simulink model "Drone_simulation"  (R2024b)
settings: Solver=VariableStepAuto  StartTime=0.0  StopTime=t_stop  RelTol=1e-3
model workspace: external: MATLAB File Drone_parameters.m (data not in the file)
values from neighbouring files (symbols this model uses):
  d = 0.20    (= 0.2)    [Drone_parameters.m]
  disturbances_enabled = 0    [Drone_parameters.m]
  flight_mode = 3    [Drone_parameters.m]
  Fx_gust = 1.0    (= 1)    [Drone_parameters.m]
  Fy_gust = 1.0    (= 1)    [Drone_parameters.m]
  Fz_gust = 0.5    [Drone_parameters.m]
  inv_m = 0.3846    [Drone_parameters.m]
  Ixx = 0.05    [Drone_parameters.m]
  Iyy = 0.05    [Drone_parameters.m]
  Izz = 0.10    (= 0.1)    [Drone_parameters.m]
  Kd_phi = 0.5    [Drone_parameters.m]
  Kd_psi = 0.5    [Drone_parameters.m]
  Kd_theta = 0.28    [Drone_parameters.m]
  Kd_x = 0.16    [Drone_parameters.m]
  Kd_y = 0.16    [Drone_parameters.m]
  Kd_z = 4.5    [Drone_parameters.m]
  kf = 4.0e-5    (= 4e-05)    [Drone_parameters.m]
  Ki_phi = 0    [Drone_parameters.m]
  Ki_psi = 0    [Drone_parameters.m]
  Ki_theta = 0.28    [Drone_parameters.m]
  Ki_x = 0    [Drone_parameters.m]
  Ki_y = 0    [Drone_parameters.m]
  Ki_z = 0    [Drone_parameters.m]
  km = 1.0e-6    (= 1e-06)    [Drone_parameters.m]
  Kp_phi = 1.0    (= 1)    [Drone_parameters.m]
  Kp_psi = 1.0    (= 1)    [Drone_parameters.m]
  Kp_theta = 0.8    [Drone_parameters.m]
  Kp_x = 0.1    [Drone_parameters.m]
  Kp_y = 0.1    [Drone_parameters.m]
  Kp_z = 1.0    (= 1)    [Drone_parameters.m]
  mg = 25.5    [Drone_parameters.m]
  N_phi = 100    [Drone_parameters.m]
  N_psi = 100    [Drone_parameters.m]
  N_theta = 100    [Drone_parameters.m]
  N_x = 100    [Drone_parameters.m]
  N_y = 100    [Drone_parameters.m]
  N_z = 100    [Drone_parameters.m]
  omega_init = 399    [Drone_parameters.m]
  phi0 = 0    [Drone_parameters.m]
  phi_dot0 = 0    [Drone_parameters.m]
  phi_manual = 0    [Drone_parameters.m]
  pitch_pair_allocation = 1/(2*d)    (= 2.5)    [Drone_parameters.m]
  psi0 = 0    [Drone_parameters.m]
  psi_des = deg2rad(0)    [Drone_parameters.m]
  psi_dot0 = 0    [Drone_parameters.m]
  psi_hold = 0    [Drone_parameters.m]
  psi_manual = 0    [Drone_parameters.m]
  rad_to_deg = 180/pi    (= 57.2957795131)    [Drone_parameters.m]
  replay_collective_to_pair_thrust_N = 51.0    (= 51)    [Drone_parameters.m]
  replay_enabled = 0    [Drone_parameters.m]
  roll_motor_allocation = 1/(4*d)    (= 1.25)    [Drone_parameters.m]
  seed_phi = 104    [Drone_parameters.m]
  seed_psi = 106    [Drone_parameters.m]
  seed_theta = 105    [Drone_parameters.m]
  seed_x = 101    [Drone_parameters.m]
  seed_y = 102    [Drone_parameters.m]
  seed_z = 103    [Drone_parameters.m]
  sensor_noise_enabled = 0    [Drone_parameters.m]
  sensor_noise_tau_attitude = 0.10    (= 0.1)    [Drone_parameters.m]
  sensor_noise_tau_position = 0.20    (= 0.2)    [Drone_parameters.m]
  sensor_sample_time = 0.02    [Drone_parameters.m]
  sigma_phi = deg2rad(0.02)    [Drone_parameters.m]
  sigma_psi = deg2rad(0.05)    [Drone_parameters.m]
  sigma_theta = deg2rad(0.02)    [Drone_parameters.m]
  sigma_x = 0.002    [Drone_parameters.m]
  sigma_y = 0.002    [Drone_parameters.m]
  sigma_z = 0.001    [Drone_parameters.m]
  t_Fx_end = 11    [Drone_parameters.m]
  t_Fx_start = 10    [Drone_parameters.m]
  t_Fy_end = 16    [Drone_parameters.m]
  t_Fy_start = 15    [Drone_parameters.m]
  t_Fz_end = 21    [Drone_parameters.m]
  t_Fz_start = 20    [Drone_parameters.m]
  t_pitch_end = 30.5    [Drone_parameters.m]
  t_pitch_start = 30    [Drone_parameters.m]
  t_roll_end = 25.5    [Drone_parameters.m]
  t_roll_start = 25    [Drone_parameters.m]
  t_step_xy = 1    [Drone_parameters.m]
  t_step_yaw = 1    [Drone_parameters.m]
  t_step_z = 0    [Drone_parameters.m]
  t_yaw_end = 35.5    [Drone_parameters.m]
  t_yaw_start = 35    [Drone_parameters.m]
  tau_m = 0.05    [Drone_parameters.m]
  tau_pitch_gust = 0.01    [Drone_parameters.m]
  tau_roll_gust = 0.01    [Drone_parameters.m]
  tau_yaw_gust = 0.002    [Drone_parameters.m]
  theta0 = 0    [Drone_parameters.m]
  theta_dot0 = 0    [Drone_parameters.m]
  theta_manual = 0    [Drone_parameters.m]
  tilt_max = 0.1745    [Drone_parameters.m]
  Tmax = 12.5    [Drone_parameters.m]
  Tmin = 0    [Drone_parameters.m]
  vx0 = 0    [Drone_parameters.m]
  vy0 = 0    [Drone_parameters.m]
  vz0 = 0    [Drone_parameters.m]
  x0 = 0    [Drone_parameters.m]
  x_des = 4    [Drone_parameters.m]
  x_hold = 0    [Drone_parameters.m]
  x_manual = 0    [Drone_parameters.m]
  y0 = 0    [Drone_parameters.m]
  y_des = 2    [Drone_parameters.m]
  y_hold = 0    [Drone_parameters.m]
  y_manual = 0    [Drone_parameters.m]
  yaw_motor_allocation = kf/(4*km)    (= 10)    [Drone_parameters.m]
  z0 = 0    [Drone_parameters.m]
  z_des = 1    [Drone_parameters.m]
  z_hold = 1    [Drone_parameters.m]
  z_manual = 1    [Drone_parameters.m]
libraries: slpidlib x6
(part 1 of 2)
settings Model: Creator=shiyu  LastModifiedBy=shiyu

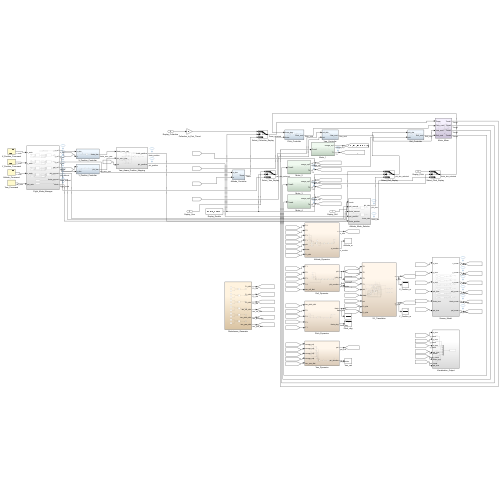
[thumbnail: Simulink's stored preview of the top-level diagram]
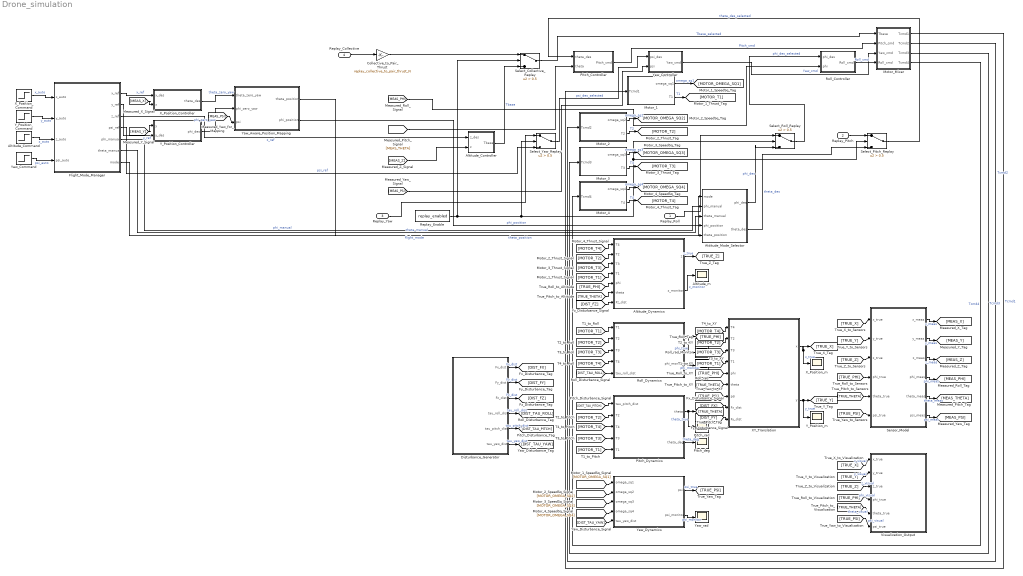
== system Drone_simulation ==
  Replay_Roll : Inport
  Replay_Pitch : Inport  Port=2
  Replay_Yaw : Inport  Port=3
  Replay_Collective : Inport  Port=4
  Altitude_Command : Step  Time=t_step_z  After=z_des  SampleTime=0
  Altitude_Controller : Subsystem  Description=Altitude error -> PID -> pair thrust correction + pair hover feed-forward. Tbase is thrust per motor pair (N).
  Altitude_Dynamics : Subsystem  Description=Inputs in unchanged port order: T4,T2,T3,T1 (N), phi,theta (rad). Both outputs are altitude (m); z_monitor duplicates z.
  Altitude_m : Scope
  Attitude_Mode_Selector : Subsystem
  Collective_to_Pair_Thrust : Gain  Gain=replay_collective_to_pair_thrust_N
  Disturbance_Generator : Subsystem  Description=Six switchable finite pulses. Outputs are world-frame forces Fx/Fy/Fz (N) and roll/pitch/yaw disturbance torques (N*m). Set disturbances_enabled=0 or 1 in Drone_parameters.m.
  Flight_Mode_Manager : Subsystem
  Motor_1 : Subsystem  Description=Motor 1: command Tcmd1 (N); output 1 omega_sq1 ((rad/s)^2), output 2 T1 (N). Rotor-speed lag and initialization preserved.
  Motor_2 : Subsystem  Description=Motor 2: command Tcmd2 (N); output 1 omega_sq2 ((rad/s)^2), output 2 T2 (N).
  Motor_3 : Subsystem  Description=Motor 3: command Tcmd3 (N); output 1 omega_sq3 ((rad/s)^2), output 2 T3 (N).
  Motor_4 : Subsystem  Description=Motor 4: command Tcmd4 (N); output 1 omega_sq4 ((rad/s)^2), output 2 T4 (N). Former Psi output was speed squared, not yaw.
  Motor_Mixer : Subsystem  Description=Input order: Tbase, Pitch_cmd, Yaw_cmd, Roll_cmd. Outputs Tcmd1..4 (N). Existing M1/M2 pair uses Tbase + Pitch_cmd; M3/M4 uses Tbase - Pitch_cmd. Do not change signs during cosmetic cleanup.
  Pitch_Controller : Subsystem  Description=Pitch angle error (rad) -> PID -> pitch pair thrust correction (N). Existing mixer sign and scaling preserved.
  Pitch_Dynamics : Subsystem  Description=Inputs: disturbance torque (N m), T2,T4,T3,T1 (N). Outputs: theta (rad), theta_deg (deg). Independent Euler-angle double integrator.
  Pitch_deg : Scope
  Pitch_rad : Scope
  Replay_Enable : Constant  Value=replay_enabled
  Roll_Controller : Subsystem  Description=Roll angle error (rad) -> PID -> per-motor differential thrust correction (N).
  Roll_Dynamics : Subsystem  Description=Inputs T1,T2,T3,T4 (N). Both outputs are roll angle (rad); phi_monitor duplicates phi. Independent Euler-angle double integrator.
  Roll_rad : Scope
  Roll_rad_Monitor : Scope
  Select_Collective_Replay : Switch  Criteria=u2 > Threshold  Threshold=0.5  SaturateOnIntegerOverflow=off  InputSameDT=off
  Select_Pitch_Replay : Switch  Criteria=u2 > Threshold  Threshold=0.5  SaturateOnIntegerOverflow=off  InputSameDT=off
  Select_Roll_Replay : Switch  Criteria=u2 > Threshold  Threshold=0.5  SaturateOnIntegerOverflow=off  InputSameDT=off
  Select_Yaw_Replay : Switch  Criteria=u2 > Threshold  Threshold=0.5  SaturateOnIntegerOverflow=off  InputSameDT=off
  Sensor_Model : Subsystem
  Visualization_Output : Subsystem
  XY_Translation : Subsystem  Description=Inputs: T4,T2,T3,T1 (N), phi,theta,psi (rad). Outputs x,y (m). Implements the ZYX body-z thrust direction: Fx/T = cos(psi)*sin(theta)*cos(phi) + sin(psi)*sin(phi); Fy/T = sin(psi)*sin(theta)*cos(phi) - cos(psi)*sin(phi). Corrected and validated 2026-09-03.
  X_Position_Command : Step  Time=t_step_xy  After=x_des  SampleTime=0
  X_Position_Controller : Subsystem  Description=x_des - x (m) -> existing PD -> pitch command limit (rad).
  X_Position_m : Scope
  Y_Position_Command : Step  Time=t_step_xy  After=y_des  SampleTime=0
  Y_Position_Controller : Subsystem  Description=Input order preserved: port 1 is actual y; port 2 is y_des. Error y_des - y, followed by existing negative roll-command sign.
  Y_Position_m : Scope
  Yaw_Aware_Position_Mapping : Subsystem
  Yaw_Command : Step  Time=t_step_yaw  After=psi_des  SampleTime=0
  Yaw_Controller : Subsystem  Description=Yaw angle error (rad) -> PID -> per-motor differential thrust correction (N).
  Yaw_Dynamics : Subsystem  Description=Inputs omega_sq1..4 ((rad/s)^2); reaction-torque coefficients are applied inside. Both outputs are yaw angle (rad); psi_monitor duplicates psi.
  Yaw_rad : Scope
  wires:
  Motor_2/1(omega_sq2) -> [MOTOR_OMEGA_SQ2]  "omega_sq2"
  Altitude_Dynamics/2(z_monitor) -> Altitude_m/1  "z_monitor"
  Roll_Dynamics/2(phi_monitor) -> Roll_rad/1  "phi_monitor"
  Yaw_Dynamics/2(psi_monitor) -> Yaw_rad/1  "psi_monitor"
  Motor_3/2(T3) -> [MOTOR_T3]  "T3"
  Pitch_Dynamics/2(theta_deg) -> Pitch_deg/1  "theta_deg"
  Motor_3/1(omega_sq3) -> [MOTOR_OMEGA_SQ3]  "omega_sq3"
  Motor_2/2(T2) -> [MOTOR_T2]  "T2"
  Flight_Mode_Manager/2(y_ref) -> Y_Position_Controller/2(y_des)  "y_ref"
  Flight_Mode_Manager/1(x_ref) -> X_Position_Controller/1(x_des)  "x_ref"
  Sensor_Model/6(psi_meas) -> [MEAS_PSI]  "psi_meas"
  Sensor_Model/5(theta_meas) -> [MEAS_THETA]  "theta_meas"
  Sensor_Model/4(phi_meas) -> [MEAS_PHI]  "phi_meas"
  Sensor_Model/3(z_meas) -> [MEAS_Z]  "z_meas"
  Sensor_Model/2(y_meas) -> [MEAS_Y]  "y_meas"
  Sensor_Model/1(x_meas) -> [MEAS_X]  "x_meas"
  Motor_4/2(T4) -> [MOTOR_T4]  "T4"
  Roll_Dynamics/1(phi) -> [TRUE_PHI], Roll_rad_Monitor/1  "phi_true"
  Pitch_Dynamics/1(theta) -> [TRUE_THETA], Pitch_rad/1  "theta_true"
  XY_Translation/1(x) -> [TRUE_X], X_Position_m/1  "x_true"
  XY_Translation/2(y) -> [TRUE_Y], Y_Position_m/1  "y_true"
  Yaw_Dynamics/1(psi) -> [TRUE_PSI]  "psi_true"
  Disturbance_Generator/1(Fx_dist) -> [DIST_FX]  "Fx_dist"
  Disturbance_Generator/2(Fy_dist) -> [DIST_FY]  "Fy_dist"
  Disturbance_Generator/3(Fz_dist) -> [DIST_FZ]  "Fz_dist"
  Disturbance_Generator/4(tau_roll_dist) -> [DIST_TAU_ROLL]  "tau_roll_dist"
  Disturbance_Generator/5(tau_pitch_dist) -> [DIST_TAU_PITCH]  "tau_pitch_dist"
  Disturbance_Generator/6(tau_yaw_dist) -> [DIST_TAU_YAW]  "tau_yaw_dist"
  X_Position_Controller/1(theta_des) -> Yaw_Aware_Position_Mapping/1(theta_zero_yaw)  "theta_zero_yaw"
  X_Position_Command/1 -> Flight_Mode_Manager/1(x_auto)  "x_auto"
  Y_Position_Controller/1(phi_des) -> Yaw_Aware_Position_Mapping/2(phi_zero_yaw)  "phi_zero_yaw"
  Y_Position_Command/1 -> Flight_Mode_Manager/2(y_auto)  "y_auto"
  Motor_4/1(omega_sq4) -> [MOTOR_OMEGA_SQ4]  "omega_sq4"
  Altitude_Dynamics/1(z) -> [TRUE_Z]  "z_true"
  Yaw_Command/1 -> Flight_Mode_Manager/4(psi_auto)  "psi_auto"
  Altitude_Command/1 -> Flight_Mode_Manager/3(z_auto)  "z_auto"
  [MEAS_X] -> X_Position_Controller/2(x)
  [MEAS_Y] -> Y_Position_Controller/1(y)
  [MOTOR_T1] -> Altitude_Dynamics/4(T1)
  [MOTOR_T2] -> Altitude_Dynamics/2(T2)
  [MOTOR_T3] -> Altitude_Dynamics/3(T3)
  [MOTOR_T4] -> Altitude_Dynamics/1(T4)
  [MOTOR_OMEGA_SQ1] -> Yaw_Dynamics/1(omega_sq1)
  [MOTOR_OMEGA_SQ2] -> Yaw_Dynamics/2(omega_sq2)
  [MOTOR_OMEGA_SQ3] -> Yaw_Dynamics/3(omega_sq3)
  [MOTOR_OMEGA_SQ4] -> Yaw_Dynamics/4(omega_sq4)
  [MEAS_PSI] -> Yaw_Aware_Position_Mapping/3(psi)
  [MOTOR_T4] -> XY_Translation/1(T4)
  [MOTOR_T4] -> Pitch_Dynamics/3(T4)
  [MOTOR_T4] -> Roll_Dynamics/4(T4)
  [MOTOR_T3] -> XY_Translation/3(T3)
  [MOTOR_T3] -> Pitch_Dynamics/4(T3)
  [MOTOR_T3] -> Roll_Dynamics/3(T3)
  [MOTOR_T2] -> XY_Translation/2(T2)
  [MOTOR_T2] -> Pitch_Dynamics/2(T2)
  [MOTOR_T2] -> Roll_Dynamics/2(T2)
  [MOTOR_T1] -> XY_Translation/4(T1)
  [MOTOR_T1] -> Pitch_Dynamics/5(T1)
  [MOTOR_T1] -> Roll_Dynamics/1(T1)
  [TRUE_X] -> Sensor_Model/1(x_true)
  [TRUE_Y] -> Sensor_Model/2(y_true)
  [TRUE_Z] -> Sensor_Model/3(z_true)
  [TRUE_PHI] -> Sensor_Model/4(phi_true)
  [TRUE_THETA] -> Sensor_Model/5(theta_true)
  [TRUE_PSI] -> Sensor_Model/6(psi_true)
  [TRUE_PHI] -> Altitude_Dynamics/5(phi)
  [TRUE_PHI] -> XY_Translation/5(phi)
  [TRUE_THETA] -> Altitude_Dynamics/6(theta)
  [TRUE_THETA] -> XY_Translation/6(theta)
  [TRUE_PSI] -> XY_Translation/7(psi)
  [DIST_FX] -> XY_Translation/8(Fx_dist)
  [DIST_FY] -> XY_Translation/9(Fy_dist)
  [DIST_FZ] -> Altitude_Dynamics/7(Fz_dist)
  [DIST_TAU_ROLL] -> Roll_Dynamics/5(tau_roll_dist)
  [DIST_TAU_PITCH] -> Pitch_Dynamics/1(tau_pitch_dist)
  [DIST_TAU_YAW] -> Yaw_Dynamics/5(tau_yaw_dist)
  [TRUE_PSI] -> Visualization_Output/6(psi_true)  "psi_visual"
  [TRUE_THETA] -> Visualization_Output/5(theta_true)  "theta_visual"
  [TRUE_PHI] -> Visualization_Output/4(phi_true)  "phi_visual"
  [TRUE_Z] -> Visualization_Output/3(z_true)  "z_visual"
  [TRUE_Y] -> Visualization_Output/2(y_true)  "y_visual"
  [TRUE_X] -> Visualization_Output/1(x_true)  "x_visual"
  Select_Collective_Replay/1 -> Motor_Mixer/1(Tbase)  "Tbase_selected"
  Altitude_Controller/1(Tbase) -> Select_Collective_Replay/3  "Tbase"
  Collective_to_Pair_Thrust/1 -> Select_Collective_Replay/1
  Replay_Collective/1 -> Collective_to_Pair_Thrust/1
  Select_Yaw_Replay/1 -> Yaw_Controller/1(psi_des)  "psi_des_selected"
  Replay_Yaw/1 -> Select_Yaw_Replay/1
  Flight_Mode_Manager/4(psi_ref) -> Select_Yaw_Replay/3  "psi_ref"
  Select_Pitch_Replay/1 -> Pitch_Controller/1(theta_des)  "theta_des_selected"
  Replay_Pitch/1 -> Select_Pitch_Replay/1
  Attitude_Mode_Selector/2(theta_des) -> Select_Pitch_Replay/3  "theta_des"
  Select_Roll_Replay/1 -> Roll_Controller/1(phi_des)  "phi_des_selected"
  Replay_Enable/1 -> Select_Pitch_Replay/2, Select_Roll_Replay/2, Select_Yaw_Replay/2, Select_Collective_Replay/2
  Replay_Roll/1 -> Select_Roll_Replay/1
  Attitude_Mode_Selector/1(phi_des) -> Select_Roll_Replay/3  "phi_des"
  [MEAS_PSI] -> Yaw_Controller/2(psi)
  [MEAS_THETA] -> Pitch_Controller/2(theta)
  [MEAS_PHI] -> Roll_Controller/2(phi)
  [MEAS_Z] -> Altitude_Controller/2(z)
  Pitch_Controller/1(Pitch_cmd) -> Motor_Mixer/2(Pitch_cmd)  "Pitch_cmd"
  Yaw_Controller/1(Yaw_cmd) -> Motor_Mixer/3(Yaw_cmd)  "Yaw_cmd"
  Motor_Mixer/4(Tcmd4) -> Motor_4/1(Tcmd4)  "Tcmd4"
  Roll_Controller/1(Roll_cmd) -> Motor_Mixer/4(Roll_cmd)  "Roll_cmd"
  Flight_Mode_Manager/3(z_ref) -> Altitude_Controller/1(z_des)  "z_ref"
  Flight_Mode_Manager/7(mode) -> Attitude_Mode_Selector/1(mode)  "flight_mode"
  Flight_Mode_Manager/5(phi_manual) -> Attitude_Mode_Selector/2(phi_manual)  "phi_manual"
  Flight_Mode_Manager/6(theta_manual) -> Attitude_Mode_Selector/3(theta_manual)  "theta_manual"
  Yaw_Aware_Position_Mapping/2(phi_position) -> Attitude_Mode_Selector/4(phi_position)  "phi_position"
  Yaw_Aware_Position_Mapping/1(theta_position) -> Attitude_Mode_Selector/5(theta_position)  "theta_position"
  Motor_Mixer/3(Tcmd3) -> Motor_3/1(Tcmd3)  "Tcmd3"
  Motor_1/2(T1) -> [MOTOR_T1]  "T1"
  Motor_Mixer/2(Tcmd2) -> Motor_2/1(Tcmd2)  "Tcmd2"
  Motor_Mixer/1(Tcmd1) -> Motor_1/1(Tcmd1)  "Tcmd1"
  Motor_1/1(omega_sq1) -> [MOTOR_OMEGA_SQ1]  "omega_sq1"

== system Drone_simulation/Altitude_Controller ==
  z_des : Inport
  z : Inport  Port=2
  Altitude_Error : Sum  Inputs=-+|
  Altitude_PID : slpidlib/PID Controller  Controller=PID  Form=Parallel  TimeDomain=Continuous-time  UseExternalTs=off  SampleTime=-1  IntegratorMethod=Forward Euler  FilterMethod=Forward Euler  ControllerParametersSource=internal  P=Kp_z  I=Ki_z  UseKiTs=off  D=Kd_z  UseExternalDerivativeSource=off  N=N_z  UseFilter=on  TunerSelectOption=Transfer Function Based (PID Tuner App)  InitialConditionSource=internal  InitialConditionForIntegrator=0  InitialConditionForFilter=0  DifferentiatorICPrevScaledInput=0  ExternalReset=none  TrackingMode=off  Kt=1  LimitOutput=off  SatLimitsSource=internal  UpperSaturationLimit=inf  LowerSaturationLimit=-inf  LinearizeAsGain=on  AntiWindupMode=none  Kb=1  LimitIntegrator=off  UpperIntegratorSaturationLimit=inf  LowerIntegratorSaturationLimit=-inf  POutMin=[]  POutMax=[]  IOutMin=[]  IOutMax=[]  DOutMin=[]  DOutMax=[]  NOutMin=[]  NOutMax=[]  SumOutMin=[]  SumOutMax=[]  SaturationOutMin=[]  SaturationOutMax=[]  PParamMin=[]  PParamMax=[]  IParamMin=[]  IParamMax=[]  DParamMin=[]  DParamMax=[]  NParamMin=[]  NParamMax=[]  KbParamMin=[]  KbParamMax=[]  KtParamMin=[]  KtParamMax=[]  KbOutMin=[]  KbOutMax=[]  KtOutMin=[]  KtOutMax=[]  IntegratorOutMin=[]  IntegratorOutMax=[]  FilterOutMin=[]  FilterOutMax=[]  SumI1OutMin=[]  SumI1OutMax=[]  SumI2OutMin=[]  SumI2OutMax=[]  SumI3OutMin=[]  SumI3OutMax=[]  SumI4OutMin=[]  SumI4OutMax=[]  SumDOutMin=[]  SumDOutMax=[]  DifferentiatorOutMin=[]  DifferentiatorOutMax=[]  FilterDiffOutCoefMin=[]  FilterDiffOutCoefMax=[]  ReciprocalOutMin=[]  ReciprocalOutMax=[]  SumDenOutMin=[]  SumDenOutMax=[]  SumNumOutMin=[]  SumNumOutMax=[]  DivideOutMin=[]  DivideOutMax=[]  UdiffTsProdOutMin=[]  UdiffTsProdOutMax=[]  NTsProdOutMin=[]  NTsProdOutMax=[]  UintegralTsProdOutMin=[]  UintegralTsProdOutMax=[]  UngainTsProdOutMin=[]  UngainTsProdOutMax=[]  ClampingZeroOutDataTypeStr=Inherit: Inherit via back propagation  ClampingZeroOutMin=[]  ClampingZeroOutMax=[]  FilterDenConstantOutDataTypeStr=Inherit: Inherit via back propagation  FilterDenConstantOutMin=[]  FilterDenConstantOutMax=[]  PCopyOutDataTypeStr=Inherit: Inherit via back propagation  PCopyOutMin=[]  PCopyOutMax=[]  NCopyOutDataTypeStr=Inherit: Inherit via back propagation  NCopyOutMin=[]  NCopyOutMax=[]  IntegratorContinuousStateAttributes=''  IntegratorStateMustResolveToSignalObject=off  IntegratorRTWStateStorageClass=Auto  FilterContinuousStateAttributes=''  FilterStateMustResolveToSignalObject=off  FilterRTWStateStorageClass=Auto  ParallelPVariant=InternalParameters  IdealPVariant=Disabled  IVariant=InternalParameters  DVariant=InternalParameters  IntegratorVariant=Continuous  SatVariant=Disabled  AWVariant=Passthrough  PCopyVariant=Disabled  TRVariant=Disabled  FdbkBlocksVariant=Forward  IdealPFdbkVariant=Disabled  SatFdbkVariant=Disabled  DerivativeFilterVariant=ContFilter  NVariant=InternalParameters  NCopyVariant=Disabled  FilterICVariant=InternalICsFilter  IntegratorICVariant=InternalICs  ExternalResetVariant=Disabled  TRSumVariant=Passthrough  SumFdbkVariant=Disabled  SumVariant=Sum_PID  TsampFilterVariant=InternalTs  TsampNgainVariant=Passthrough  TsampIntegralVariant=Disabled_SignalSpec  ExternalSaturationOutDataTypeStr=Inherit: Same as second input  DerivativeSourceVariant=ErrorSignal  PreIntVariant=InternalPreInt
  Pair_Collective_Command : Sum  Inputs=|++
  Pair_Hover_Thrust : Constant  Value=mg/2
  Total_To_Pair_Correction : Gain  Gain=0.5
  Tbase : Outport
  wires:
  z/1 -> Altitude_Error/1
  z_des/1 -> Altitude_Error/2
  Pair_Hover_Thrust/1 -> Pair_Collective_Command/2
  Pair_Collective_Command/1 -> Tbase/1
  Total_To_Pair_Correction/1 -> Pair_Collective_Command/1
  Altitude_PID/1 -> Total_To_Pair_Correction/1
  Altitude_Error/1 -> Altitude_PID/1

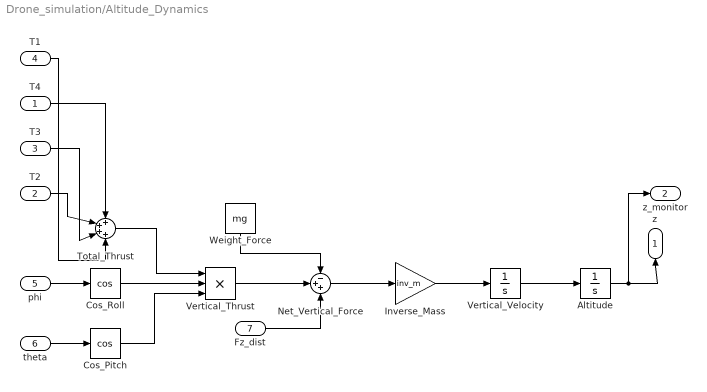
== system Drone_simulation/Altitude_Dynamics ==
  T4 : Inport
  T2 : Inport  Port=2
  T3 : Inport  Port=3
  T1 : Inport  Port=4
  phi : Inport  Port=5
  theta : Inport  Port=6
  Fz_dist : Inport  Port=7
  Altitude : Integrator  InitialCondition=z0
  Cos_Pitch : Trigonometry  Operator=cos
  Cos_Roll : Trigonometry  Operator=cos
  Inverse_Mass : Gain  Gain=inv_m
  Net_Vertical_Force : Sum  Inputs=-++
  Total_Thrust : Sum  Inputs=++++
  Vertical_Thrust : Product  Inputs=3
  Vertical_Velocity : Integrator  InitialCondition=vz0
  Weight_Force : Constant  Value=mg
  z : Outport
  z_monitor : Outport  Port=2
  wires:
  T1/1 -> Total_Thrust/4
  T2/1 -> Total_Thrust/2
  theta/1 -> Cos_Pitch/1
  Weight_Force/1 -> Net_Vertical_Force/1
  T4/1 -> Total_Thrust/1
  T3/1 -> Total_Thrust/3
  phi/1 -> Cos_Roll/1
  Total_Thrust/1 -> Vertical_Thrust/1
  Cos_Roll/1 -> Vertical_Thrust/2
  Cos_Pitch/1 -> Vertical_Thrust/3
  Altitude/1 -> z_monitor/1, z/1
  Vertical_Thrust/1 -> Net_Vertical_Force/2
  Net_Vertical_Force/1 -> Inverse_Mass/1
  Inverse_Mass/1 -> Vertical_Velocity/1
  Vertical_Velocity/1 -> Altitude/1
  Fz_dist/1 -> Net_Vertical_Force/3

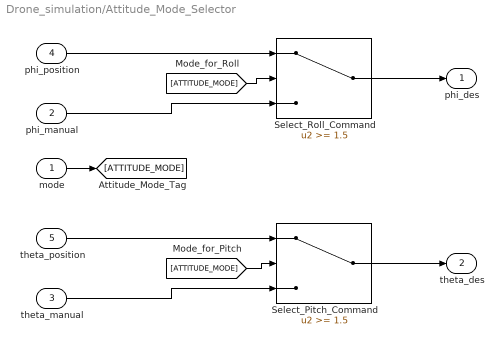
== system Drone_simulation/Attitude_Mode_Selector ==
  mode : Inport
  phi_manual : Inport  Port=2
  theta_manual : Inport  Port=3
  phi_position : Inport  Port=4
  theta_position : Inport  Port=5
  Select_Pitch_Command : Switch  Threshold=1.5  SaturateOnIntegerOverflow=off  InputSameDT=off
  Select_Roll_Command : Switch  Threshold=1.5  SaturateOnIntegerOverflow=off  InputSameDT=off
  phi_des : Outport
  theta_des : Outport  Port=2
  wires:
  [ATTITUDE_MODE] -> Select_Pitch_Command/2
  [ATTITUDE_MODE] -> Select_Roll_Command/2
  phi_position/1 -> Select_Roll_Command/1
  mode/1 -> [ATTITUDE_MODE]
  phi_manual/1 -> Select_Roll_Command/3
  Select_Roll_Command/1 -> phi_des/1
  theta_position/1 -> Select_Pitch_Command/1
  theta_manual/1 -> Select_Pitch_Command/3
  Select_Pitch_Command/1 -> theta_des/1

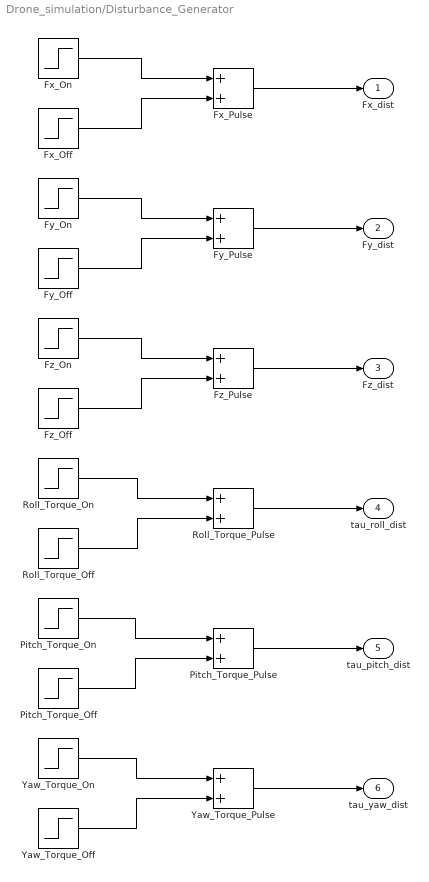
== system Drone_simulation/Disturbance_Generator ==
  Fx_Off : Step  Time=t_Fx_end  After=-disturbances_enabled*Fx_gust  SampleTime=0
  Fx_On : Step  Time=t_Fx_start  After=disturbances_enabled*Fx_gust  SampleTime=0
  Fx_Pulse : Sum
  Fy_Off : Step  Time=t_Fy_end  After=-disturbances_enabled*Fy_gust  SampleTime=0
  Fy_On : Step  Time=t_Fy_start  After=disturbances_enabled*Fy_gust  SampleTime=0
  Fy_Pulse : Sum
  Fz_Off : Step  Time=t_Fz_end  After=-disturbances_enabled*Fz_gust  SampleTime=0
  Fz_On : Step  Time=t_Fz_start  After=disturbances_enabled*Fz_gust  SampleTime=0
  Fz_Pulse : Sum
  Pitch_Torque_Off : Step  Time=t_pitch_end  After=-disturbances_enabled*tau_pitch_gust  SampleTime=0
  Pitch_Torque_On : Step  Time=t_pitch_start  After=disturbances_enabled*tau_pitch_gust  SampleTime=0
  Pitch_Torque_Pulse : Sum
  Roll_Torque_Off : Step  Time=t_roll_end  After=-disturbances_enabled*tau_roll_gust  SampleTime=0
  Roll_Torque_On : Step  Time=t_roll_start  After=disturbances_enabled*tau_roll_gust  SampleTime=0
  Roll_Torque_Pulse : Sum
  Yaw_Torque_Off : Step  Time=t_yaw_end  After=-disturbances_enabled*tau_yaw_gust  SampleTime=0
  Yaw_Torque_On : Step  Time=t_yaw_start  After=disturbances_enabled*tau_yaw_gust  SampleTime=0
  Yaw_Torque_Pulse : Sum
  Fx_dist : Outport
  Fy_dist : Outport  Port=2
  Fz_dist : Outport  Port=3
  tau_roll_dist : Outport  Port=4
  tau_pitch_dist : Outport  Port=5
  tau_yaw_dist : Outport  Port=6
  wires:
  Yaw_Torque_Pulse/1 -> tau_yaw_dist/1
  Yaw_Torque_Off/1 -> Yaw_Torque_Pulse/2
  Yaw_Torque_On/1 -> Yaw_Torque_Pulse/1
  Pitch_Torque_Pulse/1 -> tau_pitch_dist/1
  Pitch_Torque_Off/1 -> Pitch_Torque_Pulse/2
  Pitch_Torque_On/1 -> Pitch_Torque_Pulse/1
  Roll_Torque_Pulse/1 -> tau_roll_dist/1
  Roll_Torque_Off/1 -> Roll_Torque_Pulse/2
  Roll_Torque_On/1 -> Roll_Torque_Pulse/1
  Fz_Pulse/1 -> Fz_dist/1
  Fz_Off/1 -> Fz_Pulse/2
  Fz_On/1 -> Fz_Pulse/1
  Fy_Pulse/1 -> Fy_dist/1
  Fy_Off/1 -> Fy_Pulse/2
  Fy_On/1 -> Fy_Pulse/1
  Fx_Pulse/1 -> Fx_dist/1
  Fx_Off/1 -> Fx_Pulse/2
  Fx_On/1 -> Fx_Pulse/1

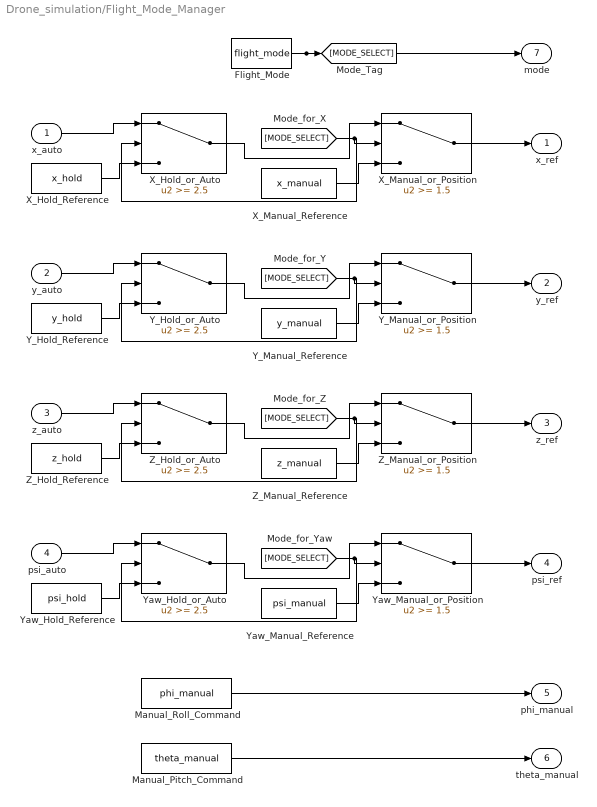
== system Drone_simulation/Flight_Mode_Manager ==
  x_auto : Inport
  y_auto : Inport  Port=2
  z_auto : Inport  Port=3
  psi_auto : Inport  Port=4
  Flight_Mode : Constant  Value=flight_mode
  Manual_Pitch_Command : Constant  Value=theta_manual
  Manual_Roll_Command : Constant  Value=phi_manual
  X_Hold_Reference : Constant  Value=x_hold
  X_Hold_or_Auto : Switch  Threshold=2.5  SaturateOnIntegerOverflow=off  InputSameDT=off
  X_Manual_Reference : Constant  Value=x_manual
  X_Manual_or_Position : Switch  Threshold=1.5  SaturateOnIntegerOverflow=off  InputSameDT=off
  Y_Hold_Reference : Constant  Value=y_hold
  Y_Hold_or_Auto : Switch  Threshold=2.5  SaturateOnIntegerOverflow=off  InputSameDT=off
  Y_Manual_Reference : Constant  Value=y_manual
  Y_Manual_or_Position : Switch  Threshold=1.5  SaturateOnIntegerOverflow=off  InputSameDT=off
  Yaw_Hold_Reference : Constant  Value=psi_hold
  Yaw_Hold_or_Auto : Switch  Threshold=2.5  SaturateOnIntegerOverflow=off  InputSameDT=off
  Yaw_Manual_Reference : Constant  Value=psi_manual
  Yaw_Manual_or_Position : Switch  Threshold=1.5  SaturateOnIntegerOverflow=off  InputSameDT=off
  Z_Hold_Reference : Constant  Value=z_hold
  Z_Hold_or_Auto : Switch  Threshold=2.5  SaturateOnIntegerOverflow=off  InputSameDT=off
  Z_Manual_Reference : Constant  Value=z_manual
  Z_Manual_or_Position : Switch  Threshold=1.5  SaturateOnIntegerOverflow=off  InputSameDT=off
  x_ref : Outport
  y_ref : Outport  Port=2
  z_ref : Outport  Port=3
  psi_ref : Outport  Port=4
  phi_manual : Outport  Port=5
  theta_manual : Outport  Port=6
  mode : Outport  Port=7
  wires:
  [MODE_SELECT] -> Yaw_Hold_or_Auto/2, Yaw_Manual_or_Position/2
  [MODE_SELECT] -> Z_Hold_or_Auto/2, Z_Manual_or_Position/2
  [MODE_SELECT] -> Y_Hold_or_Auto/2, Y_Manual_or_Position/2
  [MODE_SELECT] -> X_Hold_or_Auto/2, X_Manual_or_Position/2
  x_auto/1 -> X_Hold_or_Auto/1
  Flight_Mode/1 -> mode/1, [MODE_SELECT]
  X_Hold_Reference/1 -> X_Hold_or_Auto/3
  X_Hold_or_Auto/1 -> X_Manual_or_Position/1
  X_Manual_Reference/1 -> X_Manual_or_Position/3
  X_Manual_or_Position/1 -> x_ref/1
  y_auto/1 -> Y_Hold_or_Auto/1
  Y_Hold_Reference/1 -> Y_Hold_or_Auto/3
  Y_Hold_or_Auto/1 -> Y_Manual_or_Position/1
  Y_Manual_Reference/1 -> Y_Manual_or_Position/3
  Y_Manual_or_Position/1 -> y_ref/1
  z_auto/1 -> Z_Hold_or_Auto/1
  Z_Hold_Reference/1 -> Z_Hold_or_Auto/3
  Z_Hold_or_Auto/1 -> Z_Manual_or_Position/1
  Z_Manual_Reference/1 -> Z_Manual_or_Position/3
  Z_Manual_or_Position/1 -> z_ref/1
  psi_auto/1 -> Yaw_Hold_or_Auto/1
  Yaw_Hold_Reference/1 -> Yaw_Hold_or_Auto/3
  Yaw_Hold_or_Auto/1 -> Yaw_Manual_or_Position/1
  Yaw_Manual_Reference/1 -> Yaw_Manual_or_Position/3
  Yaw_Manual_or_Position/1 -> psi_ref/1
  Manual_Roll_Command/1 -> phi_manual/1
  Manual_Pitch_Command/1 -> theta_manual/1

== system Drone_simulation/Motor_1 ==
  Tcmd1 : Inport
  Commanded_Rotor_Speed : Sqrt
  Inverse_Motor_Time_Constant : Gain  Gain=1/tau_m
  Inverse_Thrust_Coefficient : Gain  Gain=1/kf
  Rotor_Speed : Integrator  InitialCondition=omega_init
  Rotor_Speed_Error : Sum  Inputs=|+-
  Rotor_Speed_Squared : Math  Operator=square
  Thrust_Coefficient : Gain  Gain=kf
  Thrust_Limit : Saturate  UpperLimit=Tmax  LowerLimit=Tmin
  omega_sq1 : Outport
  T1 : Outport  Port=2
  wires:
  Tcmd1/1 -> Thrust_Limit/1
  Rotor_Speed/1 -> Rotor_Speed_Error/2, Rotor_Speed_Squared/1
  Inverse_Motor_Time_Constant/1 -> Rotor_Speed/1
  Inverse_Thrust_Coefficient/1 -> Commanded_Rotor_Speed/1
  Rotor_Speed_Error/1 -> Inverse_Motor_Time_Constant/1
  Rotor_Speed_Squared/1 -> Thrust_Coefficient/1, omega_sq1/1
  Commanded_Rotor_Speed/1 -> Rotor_Speed_Error/1
  Thrust_Limit/1 -> Inverse_Thrust_Coefficient/1
  Thrust_Coefficient/1 -> T1/1

== system Drone_simulation/Motor_2 ==
  Tcmd2 : Inport
  Commanded_Rotor_Speed : Sqrt
  Inverse_Motor_Time_Constant : Gain  Gain=1/tau_m
  Inverse_Thrust_Coefficient : Gain  Gain=1/kf
  Rotor_Speed : Integrator  InitialCondition=omega_init
  Rotor_Speed_Error : Sum  Inputs=|+-
  Rotor_Speed_Squared : Math  Operator=square
  Thrust_Coefficient : Gain  Gain=kf
  Thrust_Limit : Saturate  UpperLimit=Tmax  LowerLimit=Tmin
  omega_sq2 : Outport
  T2 : Outport  Port=2
  wires:
  Tcmd2/1 -> Thrust_Limit/1
  Rotor_Speed/1 -> Rotor_Speed_Error/2, Rotor_Speed_Squared/1
  Inverse_Motor_Time_Constant/1 -> Rotor_Speed/1
  Inverse_Thrust_Coefficient/1 -> Commanded_Rotor_Speed/1
  Rotor_Speed_Squared/1 -> omega_sq2/1, Thrust_Coefficient/1
  Commanded_Rotor_Speed/1 -> Rotor_Speed_Error/1
  Rotor_Speed_Error/1 -> Inverse_Motor_Time_Constant/1
  Thrust_Limit/1 -> Inverse_Thrust_Coefficient/1
  Thrust_Coefficient/1 -> T2/1

== system Drone_simulation/Motor_3 ==
  Tcmd3 : Inport
  Commanded_Rotor_Speed : Sqrt
  Inverse_Motor_Time_Constant : Gain  Gain=1/tau_m
  Inverse_Thrust_Coefficient : Gain  Gain=1/kf
  Rotor_Speed : Integrator  InitialCondition=omega_init
  Rotor_Speed_Error : Sum  Inputs=|+-
  Rotor_Speed_Squared : Math  Operator=square
  Thrust_Coefficient : Gain  Gain=kf
  Thrust_Limit : Saturate  UpperLimit=Tmax  LowerLimit=Tmin
  omega_sq3 : Outport
  T3 : Outport  Port=2
  wires:
  Rotor_Speed_Squared/1 -> omega_sq3/1, Thrust_Coefficient/1
  Rotor_Speed/1 -> Rotor_Speed_Error/2, Rotor_Speed_Squared/1
  Inverse_Motor_Time_Constant/1 -> Rotor_Speed/1
  Thrust_Coefficient/1 -> T3/1
  Rotor_Speed_Error/1 -> Inverse_Motor_Time_Constant/1
  Commanded_Rotor_Speed/1 -> Rotor_Speed_Error/1
  Inverse_Thrust_Coefficient/1 -> Commanded_Rotor_Speed/1
  Thrust_Limit/1 -> Inverse_Thrust_Coefficient/1
  Tcmd3/1 -> Thrust_Limit/1

== system Drone_simulation/Motor_4 ==
  Tcmd4 : Inport
  Commanded_Rotor_Speed : Sqrt
  Inverse_Motor_Time_Constant : Gain  Gain=1/tau_m
  Inverse_Thrust_Coefficient : Gain  Gain=1/kf
  Rotor_Speed : Integrator  InitialCondition=omega_init
  Rotor_Speed_Error : Sum  Inputs=|+-
  Rotor_Speed_Squared : Math  Operator=square
  Thrust_Coefficient : Gain  Gain=kf
  Thrust_Limit : Saturate  UpperLimit=Tmax  LowerLimit=Tmin
  omega_sq4 : Outport
  T4 : Outport  Port=2
  wires:
  Rotor_Speed/1 -> Rotor_Speed_Error/2, Rotor_Speed_Squared/1
  Inverse_Motor_Time_Constant/1 -> Rotor_Speed/1
  Inverse_Thrust_Coefficient/1 -> Commanded_Rotor_Speed/1
  Tcmd4/1 -> Thrust_Limit/1
  Rotor_Speed_Squared/1 -> omega_sq4/1, Thrust_Coefficient/1
  Rotor_Speed_Error/1 -> Inverse_Motor_Time_Constant/1
  Commanded_Rotor_Speed/1 -> Rotor_Speed_Error/1
  Thrust_Limit/1 -> Inverse_Thrust_Coefficient/1
  Thrust_Coefficient/1 -> T4/1

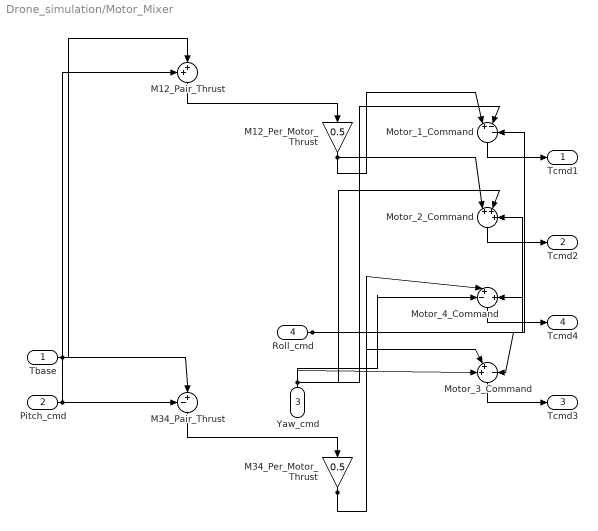
== system Drone_simulation/Motor_Mixer ==
  Tbase : Inport
  Pitch_cmd : Inport  Port=2
  Yaw_cmd : Inport  Port=3
  Roll_cmd : Inport  Port=4
  M12_Pair_Thrust : Sum  Inputs=++|
  M12_Per_Motor_Thrust : Gain  Gain=0.5
  M34_Pair_Thrust : Sum  Inputs=-+|
  M34_Per_Motor_Thrust : Gain  Gain=0.5
  Motor_1_Command : Sum  Inputs=|+--
  Motor_2_Command : Sum  Inputs=|+++
  Motor_3_Command : Sum  Inputs=++|-
  Motor_4_Command : Sum  Inputs=-+|+
  Tcmd1 : Outport
  Tcmd2 : Outport  Port=2
  Tcmd3 : Outport  Port=3
  Tcmd4 : Outport  Port=4
  wires:
  M34_Per_Motor_Thrust/1 -> Motor_4_Command/2, Motor_3_Command/2
  Yaw_cmd/1 -> Motor_1_Command/2, Motor_2_Command/2, Motor_3_Command/1, Motor_4_Command/1
  Roll_cmd/1 -> Motor_4_Command/3, Motor_3_Command/3, Motor_2_Command/3, Motor_1_Command/3
  M12_Per_Motor_Thrust/1 -> Motor_2_Command/1, Motor_1_Command/1
  Pitch_cmd/1 -> M12_Pair_Thrust/1, M34_Pair_Thrust/1
  Motor_1_Command/1 -> Tcmd1/1
  Tbase/1 -> M34_Pair_Thrust/2, M12_Pair_Thrust/2
  M34_Pair_Thrust/1 -> M34_Per_Motor_Thrust/1
  M12_Pair_Thrust/1 -> M12_Per_Motor_Thrust/1
  Motor_2_Command/1 -> Tcmd2/1
  Motor_4_Command/1 -> Tcmd4/1
  Motor_3_Command/1 -> Tcmd3/1

== system Drone_simulation/Pitch_Controller ==
  theta_des : Inport
  theta : Inport  Port=2
  Pitch_Error : Sum  Inputs=|+-
  Pitch_PID : slpidlib/PID Controller  Controller=PID  Form=Parallel  TimeDomain=Continuous-time  UseExternalTs=off  SampleTime=-1  IntegratorMethod=Forward Euler  FilterMethod=Forward Euler  ControllerParametersSource=internal  P=Kp_theta  I=Ki_theta  UseKiTs=off  D=Kd_theta  UseExternalDerivativeSource=off  N=N_theta  UseFilter=on  TunerSelectOption=Transfer Function Based (PID Tuner App)  InitialConditionSource=internal  InitialConditionForIntegrator=0  InitialConditionForFilter=0  DifferentiatorICPrevScaledInput=0  ExternalReset=none  TrackingMode=off  Kt=1  LimitOutput=off  SatLimitsSource=internal  UpperSaturationLimit=inf  LowerSaturationLimit=-inf  LinearizeAsGain=on  AntiWindupMode=none  Kb=1  LimitIntegrator=off  UpperIntegratorSaturationLimit=inf  LowerIntegratorSaturationLimit=-inf  POutMin=[]  POutMax=[]  IOutMin=[]  IOutMax=[]  DOutMin=[]  DOutMax=[]  NOutMin=[]  NOutMax=[]  SumOutMin=[]  SumOutMax=[]  SaturationOutMin=[]  SaturationOutMax=[]  PParamMin=[]  PParamMax=[]  IParamMin=[]  IParamMax=[]  DParamMin=[]  DParamMax=[]  NParamMin=[]  NParamMax=[]  KbParamMin=[]  KbParamMax=[]  KtParamMin=[]  KtParamMax=[]  KbOutMin=[]  KbOutMax=[]  KtOutMin=[]  KtOutMax=[]  IntegratorOutMin=[]  IntegratorOutMax=[]  FilterOutMin=[]  FilterOutMax=[]  SumI1OutMin=[]  SumI1OutMax=[]  SumI2OutMin=[]  SumI2OutMax=[]  SumI3OutMin=[]  SumI3OutMax=[]  SumI4OutMin=[]  SumI4OutMax=[]  SumDOutMin=[]  SumDOutMax=[]  DifferentiatorOutMin=[]  DifferentiatorOutMax=[]  FilterDiffOutCoefMin=[]  FilterDiffOutCoefMax=[]  ReciprocalOutMin=[]  ReciprocalOutMax=[]  SumDenOutMin=[]  SumDenOutMax=[]  SumNumOutMin=[]  SumNumOutMax=[]  DivideOutMin=[]  DivideOutMax=[]  UdiffTsProdOutMin=[]  UdiffTsProdOutMax=[]  NTsProdOutMin=[]  NTsProdOutMax=[]  UintegralTsProdOutMin=[]  UintegralTsProdOutMax=[]  UngainTsProdOutMin=[]  UngainTsProdOutMax=[]  ClampingZeroOutDataTypeStr=Inherit: Inherit via back propagation  ClampingZeroOutMin=[]  ClampingZeroOutMax=[]  FilterDenConstantOutDataTypeStr=Inherit: Inherit via back propagation  FilterDenConstantOutMin=[]  FilterDenConstantOutMax=[]  PCopyOutDataTypeStr=Inherit: Inherit via back propagation  PCopyOutMin=[]  PCopyOutMax=[]  NCopyOutDataTypeStr=Inherit: Inherit via back propagation  NCopyOutMin=[]  NCopyOutMax=[]  IntegratorContinuousStateAttributes=''  IntegratorStateMustResolveToSignalObject=off  IntegratorRTWStateStorageClass=Auto  FilterContinuousStateAttributes=''  FilterStateMustResolveToSignalObject=off  FilterRTWStateStorageClass=Auto  ParallelPVariant=InternalParameters  IdealPVariant=Disabled  IVariant=InternalParameters  DVariant=InternalParameters  IntegratorVariant=Continuous  SatVariant=Disabled  AWVariant=Passthrough  PCopyVariant=Disabled  TRVariant=Disabled  FdbkBlocksVariant=Forward  IdealPFdbkVariant=Disabled  SatFdbkVariant=Disabled  DerivativeFilterVariant=ContFilter  NVariant=InternalParameters  NCopyVariant=Disabled  FilterICVariant=InternalICsFilter  IntegratorICVariant=InternalICs  ExternalResetVariant=Disabled  TRSumVariant=Passthrough  SumFdbkVariant=Disabled  SumVariant=Sum_PID  TsampFilterVariant=InternalTs  TsampNgainVariant=Passthrough  TsampIntegralVariant=Disabled_SignalSpec  ExternalSaturationOutDataTypeStr=Inherit: Same as second input  DerivativeSourceVariant=ErrorSignal  PreIntVariant=InternalPreInt
  Pitch_Pair_Allocation : Gain  Gain=pitch_pair_allocation
  Pitch_cmd : Outport
  wires:
  Pitch_Pair_Allocation/1 -> Pitch_cmd/1
  Pitch_PID/1 -> Pitch_Pair_Allocation/1
  Pitch_Error/1 -> Pitch_PID/1
  theta/1 -> Pitch_Error/2
  theta_des/1 -> Pitch_Error/1

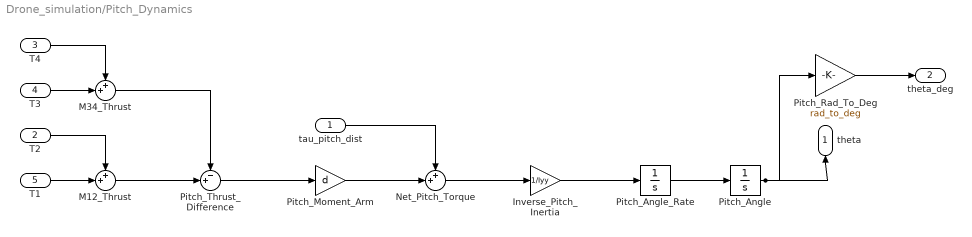
== system Drone_simulation/Pitch_Dynamics ==
  tau_pitch_dist : Inport
  T2 : Inport  Port=2
  T4 : Inport  Port=3
  T3 : Inport  Port=4
  T1 : Inport  Port=5
  Inverse_Pitch_Inertia : Gain  Gain=1/Iyy
  M12_Thrust : Sum  Inputs=++|
  M34_Thrust : Sum  Inputs=++|
  Net_Pitch_Torque : Sum  Inputs=++|
  Pitch_Angle : Integrator  InitialCondition=theta0
  Pitch_Angle_Rate : Integrator  InitialCondition=theta_dot0
  Pitch_Moment_Arm : Gain  Gain=d
  Pitch_Rad_To_Deg : Gain  Gain=rad_to_deg
  Pitch_Thrust_Difference : Sum  Inputs=-+|
  theta : Outport
  theta_deg : Outport  Port=2
  wires:
  Pitch_Angle/1 -> Pitch_Rad_To_Deg/1, theta/1
  Pitch_Thrust_Difference/1 -> Pitch_Moment_Arm/1
  T1/1 -> M12_Thrust/2
  T2/1 -> M12_Thrust/1
  Pitch_Rad_To_Deg/1 -> theta_deg/1
  T3/1 -> M34_Thrust/2
  Pitch_Angle_Rate/1 -> Pitch_Angle/1
  T4/1 -> M34_Thrust/1
  M12_Thrust/1 -> Pitch_Thrust_Difference/2
  M34_Thrust/1 -> Pitch_Thrust_Difference/1
  tau_pitch_dist/1 -> Net_Pitch_Torque/1
  Pitch_Moment_Arm/1 -> Net_Pitch_Torque/2
  Inverse_Pitch_Inertia/1 -> Pitch_Angle_Rate/1
  Net_Pitch_Torque/1 -> Inverse_Pitch_Inertia/1

== system Drone_simulation/Roll_Controller ==
  phi_des : Inport
  phi : Inport  Port=2
  Roll_Error : Sum  Inputs=|+-
  Roll_Motor_Allocation : Gain  Gain=roll_motor_allocation
  Roll_PID : slpidlib/PID Controller  Controller=PID  Form=Parallel  TimeDomain=Continuous-time  UseExternalTs=off  SampleTime=-1  IntegratorMethod=Forward Euler  FilterMethod=Forward Euler  ControllerParametersSource=internal  P=Kp_phi  I=Ki_phi  UseKiTs=off  D=Kd_phi  UseExternalDerivativeSource=off  N=N_phi  UseFilter=on  TunerSelectOption=Transfer Function Based (PID Tuner App)  InitialConditionSource=internal  InitialConditionForIntegrator=0  InitialConditionForFilter=0  DifferentiatorICPrevScaledInput=0  ExternalReset=none  TrackingMode=off  Kt=1  LimitOutput=off  SatLimitsSource=internal  UpperSaturationLimit=inf  LowerSaturationLimit=-inf  LinearizeAsGain=on  AntiWindupMode=none  Kb=1  LimitIntegrator=off  UpperIntegratorSaturationLimit=inf  LowerIntegratorSaturationLimit=-inf  POutMin=[]  POutMax=[]  IOutMin=[]  IOutMax=[]  DOutMin=[]  DOutMax=[]  NOutMin=[]  NOutMax=[]  SumOutMin=[]  SumOutMax=[]  SaturationOutMin=[]  SaturationOutMax=[]  PParamMin=[]  PParamMax=[]  IParamMin=[]  IParamMax=[]  DParamMin=[]  DParamMax=[]  NParamMin=[]  NParamMax=[]  KbParamMin=[]  KbParamMax=[]  KtParamMin=[]  KtParamMax=[]  KbOutMin=[]  KbOutMax=[]  KtOutMin=[]  KtOutMax=[]  IntegratorOutMin=[]  IntegratorOutMax=[]  FilterOutMin=[]  FilterOutMax=[]  SumI1OutMin=[]  SumI1OutMax=[]  SumI2OutMin=[]  SumI2OutMax=[]  SumI3OutMin=[]  SumI3OutMax=[]  SumI4OutMin=[]  SumI4OutMax=[]  SumDOutMin=[]  SumDOutMax=[]  DifferentiatorOutMin=[]  DifferentiatorOutMax=[]  FilterDiffOutCoefMin=[]  FilterDiffOutCoefMax=[]  ReciprocalOutMin=[]  ReciprocalOutMax=[]  SumDenOutMin=[]  SumDenOutMax=[]  SumNumOutMin=[]  SumNumOutMax=[]  DivideOutMin=[]  DivideOutMax=[]  UdiffTsProdOutMin=[]  UdiffTsProdOutMax=[]  NTsProdOutMin=[]  NTsProdOutMax=[]  UintegralTsProdOutMin=[]  UintegralTsProdOutMax=[]  UngainTsProdOutMin=[]  UngainTsProdOutMax=[]  ClampingZeroOutDataTypeStr=Inherit: Inherit via back propagation  ClampingZeroOutMin=[]  ClampingZeroOutMax=[]  FilterDenConstantOutDataTypeStr=Inherit: Inherit via back propagation  FilterDenConstantOutMin=[]  FilterDenConstantOutMax=[]  PCopyOutDataTypeStr=Inherit: Inherit via back propagation  PCopyOutMin=[]  PCopyOutMax=[]  NCopyOutDataTypeStr=Inherit: Inherit via back propagation  NCopyOutMin=[]  NCopyOutMax=[]  IntegratorContinuousStateAttributes=''  IntegratorStateMustResolveToSignalObject=off  IntegratorRTWStateStorageClass=Auto  FilterContinuousStateAttributes=''  FilterStateMustResolveToSignalObject=off  FilterRTWStateStorageClass=Auto  ParallelPVariant=InternalParameters  IdealPVariant=Disabled  IVariant=InternalParameters  DVariant=InternalParameters  IntegratorVariant=Continuous  SatVariant=Disabled  AWVariant=Passthrough  PCopyVariant=Disabled  TRVariant=Disabled  FdbkBlocksVariant=Forward  IdealPFdbkVariant=Disabled  SatFdbkVariant=Disabled  DerivativeFilterVariant=ContFilter  NVariant=InternalParameters  NCopyVariant=Disabled  FilterICVariant=InternalICsFilter  IntegratorICVariant=InternalICs  ExternalResetVariant=Disabled  TRSumVariant=Passthrough  SumFdbkVariant=Disabled  SumVariant=Sum_PID  TsampFilterVariant=InternalTs  TsampNgainVariant=Passthrough  TsampIntegralVariant=Disabled_SignalSpec  ExternalSaturationOutDataTypeStr=Inherit: Same as second input  DerivativeSourceVariant=ErrorSignal  PreIntVariant=InternalPreInt
  Roll_cmd : Outport
  wires:
  Roll_Motor_Allocation/1 -> Roll_cmd/1
  Roll_PID/1 -> Roll_Motor_Allocation/1
  Roll_Error/1 -> Roll_PID/1
  phi/1 -> Roll_Error/2
  phi_des/1 -> Roll_Error/1

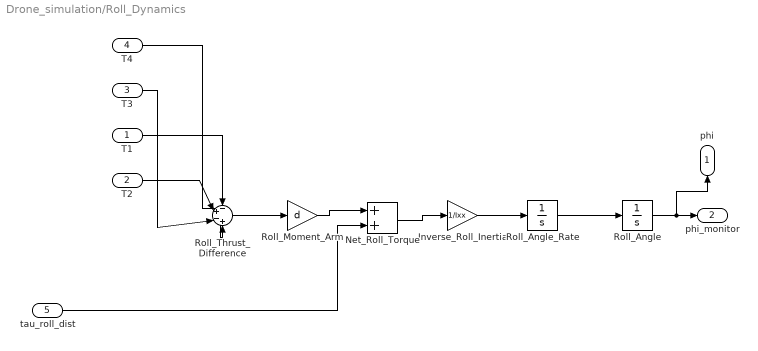
== system Drone_simulation/Roll_Dynamics ==
  T1 : Inport
  T2 : Inport  Port=2
  T3 : Inport  Port=3
  T4 : Inport  Port=4
  tau_roll_dist : Inport  Port=5
  Inverse_Roll_Inertia : Gain  Gain=1/Ixx
  Net_Roll_Torque : Sum
  Roll_Angle : Integrator  InitialCondition=phi0
  Roll_Angle_Rate : Integrator  InitialCondition=phi_dot0
  Roll_Moment_Arm : Gain  Gain=d
  Roll_Thrust_Difference : Sum  Inputs=-+-+
  phi : Outport
  phi_monitor : Outport  Port=2
  wires:
  T2/1 -> Roll_Thrust_Difference/2
  T1/1 -> Roll_Thrust_Difference/1
  T3/1 -> Roll_Thrust_Difference/3
  T4/1 -> Roll_Thrust_Difference/4
  Inverse_Roll_Inertia/1 -> Roll_Angle_Rate/1
  Net_Roll_Torque/1 -> Inverse_Roll_Inertia/1
  tau_roll_dist/1 -> Net_Roll_Torque/2
  Roll_Moment_Arm/1 -> Net_Roll_Torque/1
  Roll_Thrust_Difference/1 -> Roll_Moment_Arm/1
  Roll_Angle_Rate/1 -> Roll_Angle/1
  Roll_Angle/1 -> phi/1, phi_monitor/1

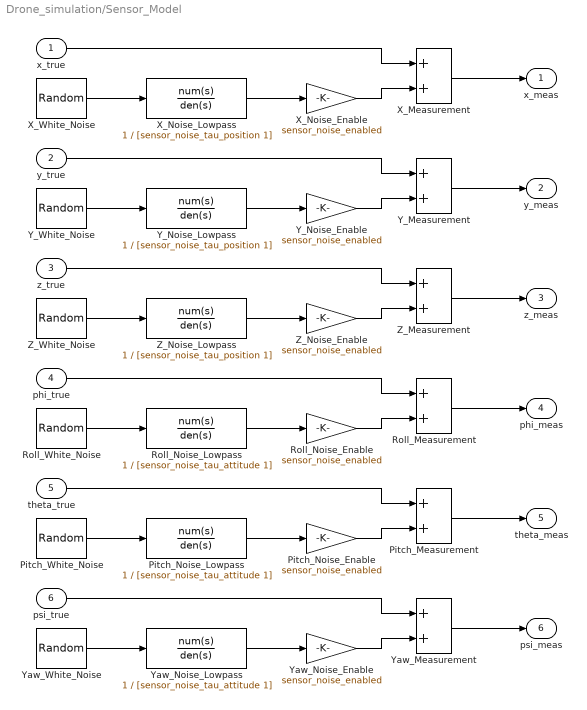
== system Drone_simulation/Sensor_Model ==
  x_true : Inport
  y_true : Inport  Port=2
  z_true : Inport  Port=3
  phi_true : Inport  Port=4
  theta_true : Inport  Port=5
  psi_true : Inport  Port=6
  Pitch_Measurement : Sum
  Pitch_Noise_Enable : Gain  Gain=sensor_noise_enabled
  Pitch_Noise_Lowpass : TransferFcn  Numerator=1  Denominator=[sensor_noise_tau_attitude 1]
  Pitch_White_Noise : RandomNumber  Variance=sigma_theta^2  Seed=seed_theta  SampleTime=sensor_sample_time
  Roll_Measurement : Sum
  Roll_Noise_Enable : Gain  Gain=sensor_noise_enabled
  Roll_Noise_Lowpass : TransferFcn  Numerator=1  Denominator=[sensor_noise_tau_attitude 1]
  Roll_White_Noise : RandomNumber  Variance=sigma_phi^2  Seed=seed_phi  SampleTime=sensor_sample_time
  X_Measurement : Sum
  X_Noise_Enable : Gain  Gain=sensor_noise_enabled
  X_Noise_Lowpass : TransferFcn  Numerator=1  Denominator=[sensor_noise_tau_position 1]
  X_White_Noise : RandomNumber  Variance=sigma_x^2  Seed=seed_x  SampleTime=sensor_sample_time
  Y_Measurement : Sum
  Y_Noise_Enable : Gain  Gain=sensor_noise_enabled
  Y_Noise_Lowpass : TransferFcn  Numerator=1  Denominator=[sensor_noise_tau_position 1]
  Y_White_Noise : RandomNumber  Variance=sigma_y^2  Seed=seed_y  SampleTime=sensor_sample_time
  Yaw_Measurement : Sum
  Yaw_Noise_Enable : Gain  Gain=sensor_noise_enabled
  Yaw_Noise_Lowpass : TransferFcn  Numerator=1  Denominator=[sensor_noise_tau_attitude 1]
  Yaw_White_Noise : RandomNumber  Variance=sigma_psi^2  Seed=seed_psi  SampleTime=sensor_sample_time
  Z_Measurement : Sum
  Z_Noise_Enable : Gain  Gain=sensor_noise_enabled
  Z_Noise_Lowpass : TransferFcn  Numerator=1  Denominator=[sensor_noise_tau_position 1]
  Z_White_Noise : RandomNumber  Variance=sigma_z^2  Seed=seed_z  SampleTime=sensor_sample_time
  x_meas : Outport
  y_meas : Outport  Port=2
  z_meas : Outport  Port=3
  phi_meas : Outport  Port=4
  theta_meas : Outport  Port=5
  psi_meas : Outport  Port=6
  wires:
  Yaw_Noise_Lowpass/1 -> Yaw_Noise_Enable/1
  Pitch_Noise_Lowpass/1 -> Pitch_Noise_Enable/1
  Roll_Noise_Lowpass/1 -> Roll_Noise_Enable/1
  Z_Noise_Lowpass/1 -> Z_Noise_Enable/1
  Y_Noise_Lowpass/1 -> Y_Noise_Enable/1
  X_Noise_Lowpass/1 -> X_Noise_Enable/1
  X_White_Noise/1 -> X_Noise_Lowpass/1
  x_true/1 -> X_Measurement/1
  X_Noise_Enable/1 -> X_Measurement/2
  X_Measurement/1 -> x_meas/1
  Y_White_Noise/1 -> Y_Noise_Lowpass/1
  y_true/1 -> Y_Measurement/1
  Y_Noise_Enable/1 -> Y_Measurement/2
  Y_Measurement/1 -> y_meas/1
  Z_White_Noise/1 -> Z_Noise_Lowpass/1
  z_true/1 -> Z_Measurement/1
  Z_Noise_Enable/1 -> Z_Measurement/2
  Z_Measurement/1 -> z_meas/1
  Roll_White_Noise/1 -> Roll_Noise_Lowpass/1
  phi_true/1 -> Roll_Measurement/1
  Roll_Noise_Enable/1 -> Roll_Measurement/2
  Roll_Measurement/1 -> phi_meas/1
  Pitch_White_Noise/1 -> Pitch_Noise_Lowpass/1
  theta_true/1 -> Pitch_Measurement/1
  Pitch_Noise_Enable/1 -> Pitch_Measurement/2
  Pitch_Measurement/1 -> theta_meas/1
  Yaw_White_Noise/1 -> Yaw_Noise_Lowpass/1
  psi_true/1 -> Yaw_Measurement/1
  Yaw_Noise_Enable/1 -> Yaw_Measurement/2
  Yaw_Measurement/1 -> psi_meas/1

== system Drone_simulation/Visualization_Output ==
  x_true : Inport
  y_true : Inport  Port=2
  z_true : Inport  Port=3
  phi_true : Inport  Port=4
  theta_true : Inport  Port=5
  psi_true : Inport  Port=6
  Flight_Visualization_Data : ToWorkspace  VariableName=flight_visualization  SaveFormat=Timeseries  SampleTime=-1
  State_Vector : Mux  Inputs=6
  wires:
  State_Vector/1 -> Flight_Visualization_Data/1  "state_3d"
  psi_true/1 -> State_Vector/6
  theta_true/1 -> State_Vector/5
  phi_true/1 -> State_Vector/4
  z_true/1 -> State_Vector/3
  y_true/1 -> State_Vector/2
  x_true/1 -> State_Vector/1

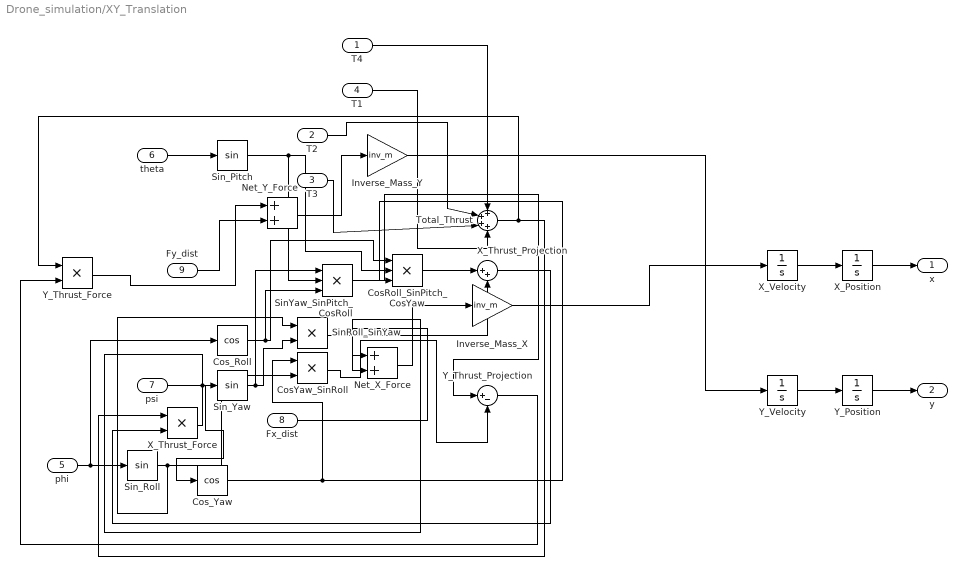
== system Drone_simulation/XY_Translation ==
  T4 : Inport
  T2 : Inport  Port=2
  T3 : Inport  Port=3
  T1 : Inport  Port=4
  phi : Inport  Port=5
  theta : Inport  Port=6
  psi : Inport  Port=7
  Fx_dist : Inport  Port=8
  Fy_dist : Inport  Port=9
  CosRoll_SinPitch_CosYaw : Product  Inputs=3
  CosYaw_SinRoll : Product
  Cos_Roll : Trigonometry  Operator=cos
  Cos_Yaw : Trigonometry  Operator=cos
  Inverse_Mass_X : Gain  Gain=inv_m
  Inverse_Mass_Y : Gain  Gain=inv_m
  Net_X_Force : Sum
  Net_Y_Force : Sum
  SinRoll_SinYaw : Product
  SinYaw_SinPitch_CosRoll : Product  Inputs=3
  Sin_Pitch : Trigonometry
  Sin_Roll : Trigonometry
  Sin_Yaw : Trigonometry
  Total_Thrust : Sum  Inputs=++++
  X_Position : Integrator  InitialCondition=x0
  X_Thrust_Force : Product
  X_Thrust_Projection : Sum  Inputs=|++
  X_Velocity : Integrator  InitialCondition=vx0
  Y_Position : Integrator  InitialCondition=y0
  Y_Thrust_Force : Product
  Y_Thrust_Projection : Sum  Inputs=|+-
  Y_Velocity : Integrator  InitialCondition=vy0
  x : Outport
  y : Outport  Port=2
  wires:
  X_Position/1 -> x/1
  T4/1 -> Total_Thrust/1
  theta/1 -> Sin_Pitch/1
  Y_Position/1 -> y/1
  T1/1 -> Total_Thrust/4
  X_Velocity/1 -> X_Position/1
  Y_Velocity/1 -> Y_Position/1
  SinYaw_SinPitch_CosRoll/1 -> Y_Thrust_Projection/1
  CosRoll_SinPitch_CosYaw/1 -> X_Thrust_Projection/1
  Sin_Pitch/1 -> SinYaw_SinPitch_CosRoll/2, CosRoll_SinPitch_CosYaw/2
  Cos_Roll/1 -> SinYaw_SinPitch_CosRoll/3, CosRoll_SinPitch_CosYaw/1
  Net_Y_Force/1 -> Inverse_Mass_Y/1
  Fy_dist/1 -> Net_Y_Force/2
  Y_Thrust_Force/1 -> Net_Y_Force/1
  Net_X_Force/1 -> Inverse_Mass_X/1
  Fx_dist/1 -> Net_X_Force/2
  X_Thrust_Force/1 -> Net_X_Force/1
  phi/1 -> Cos_Roll/1, Sin_Roll/1
  psi/1 -> Cos_Yaw/1, Sin_Yaw/1
  Sin_Roll/1 -> SinRoll_SinYaw/1, CosYaw_SinRoll/2
  Sin_Yaw/1 -> SinYaw_SinPitch_CosRoll/1, SinRoll_SinYaw/2
  Cos_Yaw/1 -> CosRoll_SinPitch_CosYaw/3, CosYaw_SinRoll/1
  CosYaw_SinRoll/1 -> Y_Thrust_Projection/2
  Inverse_Mass_X/1 -> X_Velocity/1
  Y_Thrust_Projection/1 -> Y_Thrust_Force/2
  Total_Thrust/1 -> X_Thrust_Force/1, Y_Thrust_Force/1
  SinRoll_SinYaw/1 -> X_Thrust_Projection/2
  X_Thrust_Projection/1 -> X_Thrust_Force/2
  T2/1 -> Total_Thrust/2
  Inverse_Mass_Y/1 -> Y_Velocity/1
  T3/1 -> Total_Thrust/3
